simulink model "experiment_file"  (Simulink 8.3)
settings: Solver=ode1  StartTime=0.0  StopTime=inf  FixedStep=0.01  RelTol=1e-3
values from neighbouring files (symbols this model uses):
  accuratepath = interplotation(path)    [Pathplanning.m]    (also in interplotation.m = [accuratepath;interp1([1,insertnum+2],[pathfromstartpoint(i,)
undefined symbols (not defined in the file or in its folder): HIL
libraries: quarc_library x8
settings Model: Creator=drmadill  LastModifiedBy=WXY  SimulationMode=external  ExtModeTrigDuration=1
settings SolverCC: PositivePriorityOrder=on
settings OptimizationCC: ExpressionDepthLimit=2147483647  LifeSpan=auto
settings DebuggingCC: FrameProcessingCompatibilityMsg=error
settings RTWCC: SystemTargetFile=quarc_linux_pi_3.tlc  TemplateMakefile=quarc_linux_pi_3_tmf  Description=QUARC Linux Raspberry Pi 3 Target  ProcessScript=quarc_linux_pi_3_make_rtw_hook
settings STFCustomTargetCC: TargetLibSuffix=.a  TargetPreCompLibLocation=C:\PROGRA~3\QUARC\lib\2017a\LICFC8~1\release  ConcurrentExecutionCompliant=on  SystemTargetFile=quarc_linux_pi_3.tlc
settings GRTTargetCC: TargetLibSuffix=.a  TargetPreCompLibLocation=C:\PROGRA~3\QUARC\lib\2017a\LICFC8~1\release  ParMdlRefBuildCompliant=off  CompOptLevelCompliant=off  GeneratePreprocessorConditionals=Use local settings  MatFileLogging=off  CPPClassGenCompliant=off  ExtMode=on  ExtModeMexFile=quarc_comm  ExtModeMexArgs='-w -d /tmp -uri %u'
settings ConfigComp: CovMetricSettings=dw  CovHtmlReporting=on  CovSaveCumulativeToWorkspaceVar=on  CovSaveSingleToWorkspaceVar=on  CovExternalEMLEnable=off  CovSFcnEnable=off

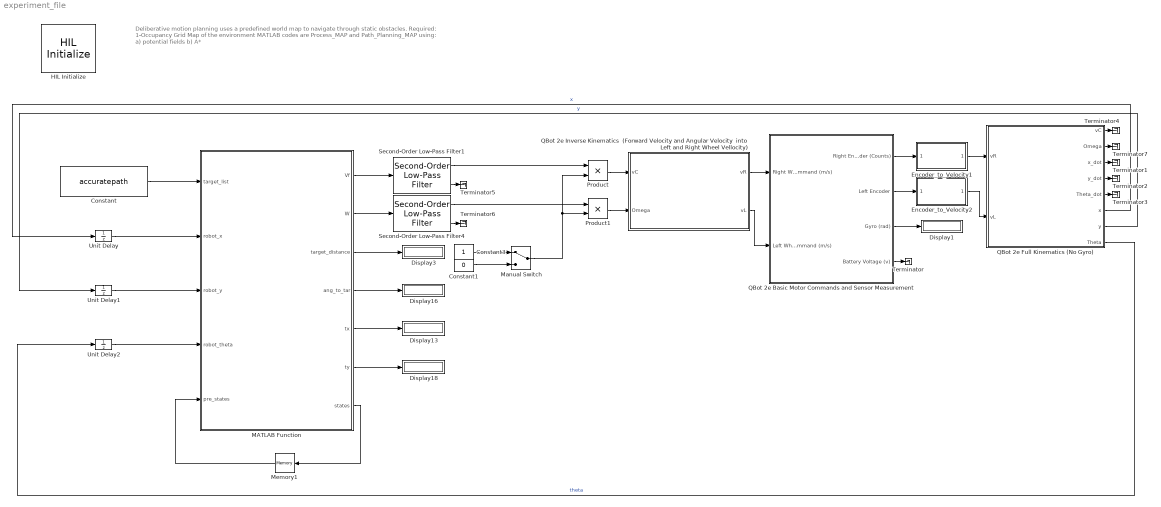
== system experiment_file ==
  note: Deliberative motion planning uses a predefined world map to navigate through static obstacles.
      |
      | Required:
      | 1-Occupancy Grid Map of the environment
      | MATLAB codes are Process_MAP and Path_Planning_MAP using:
      | a) potential fields
      | b) A*
  Constant : Constant  Value=accuratepath
  Constant1 : Constant  Value=0
  Constant3 : Constant
  Display{1,3,13,16,18} (5 alike) : Display
  Encoder_to_Velocity1 : Subsystem
  Encoder_to_Velocity2 : Subsystem
  HIL Initialize : quarc_library/Data Acquisition/Generic/Configuration/HIL Initialize  Priority=-99  object_name=HIL-1  board_type=qbot2e  board_number=0  board_options=pwm0_en=1;pwm0_pin=12;pwm1_en=1;pwm1_pin=13;  exclusive=off  active=off  hardware_clocks=[]  clock_modes=[]  initial_clock_frequencies=[]  set_clock_params_at_start=off  set_clock_params_at_switch_in=off  set_clock_frequencies_at_start=off  set_clock_frequencies_at_switch_in=off  analog_input_channels=[0:5]  analog_input_configurations=[]  analog_input_maximums=[16.5 3.3 3.3 3.3 3.3 3.3]  analog_input_minimums=[0 0 0 0 0 0]  set_analog_input_params_at_start=off  set_analog_input_params_at_switch_in=off  analog_output_channels=[]  analog_output_maximums=[]  analog_output_minimums=[]  initial_analog_outputs=[]  final_analog_outputs=[]  watchdog_analog_outputs=[]  set_analog_output_params_at_start=off  set_analog_output_params_at_switch_in=off  set_analog_outputs_at_start=off  set_analog_outputs_at_switch_in=off  set_analog_outputs_at_terminate=off  set_analog_outputs_at_switch_out=off  set_analog_outputs_on_watchdog=off  digital_input_channels=[28:58]  digital_output_channels=[28:31]  digital_output_configuration=[]  initial_digital_outputs=[0]  final_digital_outputs=[0]  watchdog_digital_outputs=[]  set_digital_output_params_at_start=off  set_digital_output_params_at_switch_in=off  set_digital_outputs_at_start=on  set_digital_outputs_at_switch_in=off  set_digital_outputs_at_terminate=on  set_digital_outputs_at_switch_out=off  set_digital_outputs_on_watchdog=off  encoder_channels=[0:1]  quadrature=[4]  encoder_filter_frequency=[]  initial_encoder_counts=[0]  set_encoder_params_at_start=on  set_encoder_params_at_switch_in=off  set_encoder_counts_at_start=on  set_encoder_counts_at_switch_in=off  pwm_channels=[0:1]  pwm_modes=0  pwm_frequency=100e6 / 4095  pwm_configuration=[0]  pwm_alignment=[0]  pwm_polarity=[1]  pwm_leading_deadband=[]  pwm_trailing_deadband=[]  initial_pwm_outputs=[0]  final_pwm_outputs=[0]  watchdog_pwm_outputs=[]  set_pwm_params_at_start=on  set_pwm_params_at_switch_in=off  set_pwm_outputs_at_start=on  set_pwm_outputs_at_switch_in=off  set_pwm_outputs_at_terminate=on  set_pwm_outputs_at_switch_out=off  set_pwm_outputs_on_watchdog=off  other_output_channels=[2000:2001 14000 16000]  initial_other_outputs=[0 0 0 7]  final_other_outputs=[0 0 0 7]  watchdog_other_outputs=[]  set_other_outputs_at_start=on  set_other_outputs_at_switch_in=off  set_other_outputs_at_terminate=on  set_other_outputs_at_switch_out=off  set_other_outputs_on_watchdog=off
  MATLAB Function : MATLAB Function  TreatAsAtomicUnit=on
  Manual Switch : ManualSwitch
  Memory1 : Memory  X0=[1]
  Product : Product  RndMeth=Zero
  Product1 : Product  RndMeth=Zero
  QBot 2e Basic Motor Commands and Sensor Measurement : Subsystem
  QBot 2e Full Kinematics (No Gyro) : Subsystem
  QBot 2e Inverse Kinematics  (Forward Velocity and Angular Velocity  into Left and Right Wheel Vellocity) : Subsystem
  Second-Order Low-Pass Filter1 : quarc_library/Continuous/Second-Order Low-Pass Filter  params_source=Internal (dialog parameters)  input_width=30  input_zeta=1  input_init=0
  Second-Order Low-Pass Filter4 : quarc_library/Continuous/Second-Order Low-Pass Filter  params_source=Internal (dialog parameters)  input_width=60  input_zeta=1  input_init=0
  Terminator{,1..7} (8 alike) : Terminator
  Unit Delay : UnitDelay  SampleTime=-1
  Unit Delay1 : UnitDelay  SampleTime=-1
  Unit Delay2 : UnitDelay  SampleTime=-1
  wires:
  Constant3/1 -> Manual Switch/1
  Constant1/1 -> Manual Switch/2
  QBot 2e Basic Motor Commands and Sensor Measurement/1(Right Encoder (Counts)) -> Encoder_to_Velocity1/1(Encoder)
  QBot 2e Basic Motor Commands and Sensor Measurement/2(Left Encoder) -> Encoder_to_Velocity2/1(Encoder)
  QBot 2e Basic Motor Commands and Sensor Measurement/3(Gyro (rad)) -> Display1/1
  Encoder_to_Velocity1/1(Velocity) -> QBot 2e Full Kinematics (No Gyro)/1(vR)
  Encoder_to_Velocity2/1(Velocity) -> QBot 2e Full Kinematics (No Gyro)/2(vL)
  Second-Order Low-Pass Filter1/1 -> Product/1
  Second-Order Low-Pass Filter4/1 -> Product1/1
  QBot 2e Inverse Kinematics  (Forward Velocity and Angular Velocity  into Left and Right Wheel Vellocity)/1(vR) -> QBot 2e Basic Motor Commands and Sensor Measurement/1(Right Wheel Command (m/s))
  QBot 2e Inverse Kinematics  (Forward Velocity and Angular Velocity  into Left and Right Wheel Vellocity)/2(vL) -> QBot 2e Basic Motor Commands and Sensor Measurement/2(Left Wheel Command (m/s))
  Product/1 -> QBot 2e Inverse Kinematics  (Forward Velocity and Angular Velocity  into Left and Right Wheel Vellocity)/1(vC)
  Product1/1 -> QBot 2e Inverse Kinematics  (Forward Velocity and Angular Velocity  into Left and Right Wheel Vellocity)/2(Omega)
  Manual Switch/1 -> Product/2, Product1/2
  QBot 2e Full Kinematics (No Gyro)/3(x_dot) -> Terminator1/1
  QBot 2e Full Kinematics (No Gyro)/4(y_dot) -> Terminator2/1
  QBot 2e Full Kinematics (No Gyro)/5(Theta_dot) -> Terminator3/1
  MATLAB Function/3(target_distance) -> Display3/1
  MATLAB Function/4(ang_to_tar) -> Display16/1
  MATLAB Function/1(Vf) -> Second-Order Low-Pass Filter1/1
  MATLAB Function/2(W) -> Second-Order Low-Pass Filter4/1
  QBot 2e Full Kinematics (No Gyro)/8(Theta) -> Unit Delay2/1  "theta"
  MATLAB Function/5(tx) -> Display13/1
  MATLAB Function/6(ty) -> Display18/1
  QBot 2e Full Kinematics (No Gyro)/6(x) -> Unit Delay/1  "x"
  QBot 2e Full Kinematics (No Gyro)/7(y) -> Unit Delay1/1  "y"
  Second-Order Low-Pass Filter1/2 -> Terminator5/1
  Second-Order Low-Pass Filter4/2 -> Terminator6/1
  QBot 2e Full Kinematics (No Gyro)/1(vC) -> Terminator4/1
  QBot 2e Full Kinematics (No Gyro)/2(Omega) -> Terminator7/1
  QBot 2e Basic Motor Commands and Sensor Measurement/4(Battery Voltage (v)) -> Terminator/1
  Constant/1 -> MATLAB Function/1(target_list)
  Unit Delay/1 -> MATLAB Function/2(robot_x)
  Unit Delay1/1 -> MATLAB Function/3(robot_y)
  Unit Delay2/1 -> MATLAB Function/4(robot_theta)
  MATLAB Function/7(states) -> Memory1/1
  Memory1/1 -> MATLAB Function/5(pre_states)

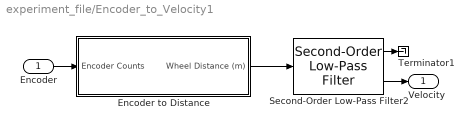
== system experiment_file/Encoder_to_Velocity1 ==
  Encoder : Inport
  Encoder to Distance : Subsystem
  Second-Order Low-Pass Filter2 : quarc_library/Continuous/Second-Order Low-Pass Filter  params_source=Internal (dialog parameters)  input_width=10  input_zeta=1  input_init=0
  Terminator1 : Terminator
  Velocity : Outport
  wires:
  Second-Order Low-Pass Filter2/1 -> Terminator1/1
  Encoder to Distance/1(Wheel Distance (m)) -> Second-Order Low-Pass Filter2/1
  Encoder/1 -> Encoder to Distance/1(Encoder Counts)
  Second-Order Low-Pass Filter2/2 -> Velocity/1

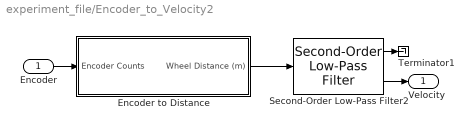
== system experiment_file/Encoder_to_Velocity2 ==
  Encoder : Inport
  Encoder to Distance : Subsystem
  Second-Order Low-Pass Filter2 : quarc_library/Continuous/Second-Order Low-Pass Filter  params_source=Internal (dialog parameters)  input_width=10  input_zeta=1  input_init=0
  Terminator1 : Terminator
  Velocity : Outport
  wires:
  Second-Order Low-Pass Filter2/2 -> Velocity/1
  Encoder/1 -> Encoder to Distance/1(Encoder Counts)
  Encoder to Distance/1(Wheel Distance (m)) -> Second-Order Low-Pass Filter2/1
  Second-Order Low-Pass Filter2/1 -> Terminator1/1

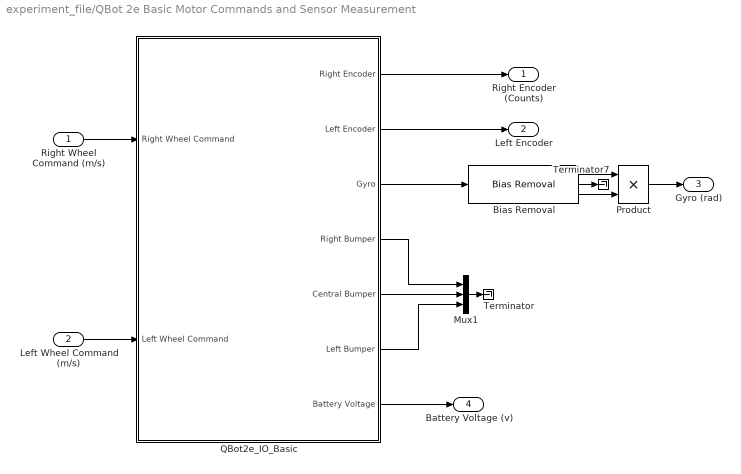
== system experiment_file/QBot 2e Basic Motor Commands and Sensor Measurement ==
  Right Wheel Command (m/s) : Inport
  Left Wheel Command (m/s) : Inport  Port=2
  Bias Removal : quarc_library/Discrete/Bias Removal  start_time=3  end_time=4  switch_id=0  sample_time=qc_get_step_size
      settings: SourceProductName=QUARC Targets
  Mux1 : Mux  Inputs=3
  Product : Product  RndMeth=Zero
  QBot2e_IO_Basic : Subsystem
  Terminator : Terminator
  Terminator7 : Terminator
  Right Encoder (Counts) : Outport
  Left Encoder : Outport  Port=2
  Gyro (rad) : Outport  Port=3
  Battery Voltage (v) : Outport  Port=4
  wires:
  QBot2e_IO_Basic/4(Right Bumper) -> Mux1/1
  QBot2e_IO_Basic/5(Central Bumper) -> Mux1/2
  QBot2e_IO_Basic/6(Left Bumper) -> Mux1/3
  Right Wheel Command (m/s)/1 -> QBot2e_IO_Basic/1(Right Wheel Command)
  Left Wheel Command (m/s)/1 -> QBot2e_IO_Basic/2(Left Wheel Command)
  QBot2e_IO_Basic/1(Right Encoder) -> Right Encoder (Counts)/1
  QBot2e_IO_Basic/2(Left Encoder) -> Left Encoder/1
  QBot2e_IO_Basic/7(Battery Voltage) -> Battery Voltage (v)/1
  Bias Removal/2 -> Terminator7/1
  Bias Removal/1 -> Product/1
  Bias Removal/3 -> Product/2
  Product/1 -> Gyro (rad)/1
  QBot2e_IO_Basic/3(Gyro) -> Bias Removal/1
  Mux1/1 -> Terminator/1

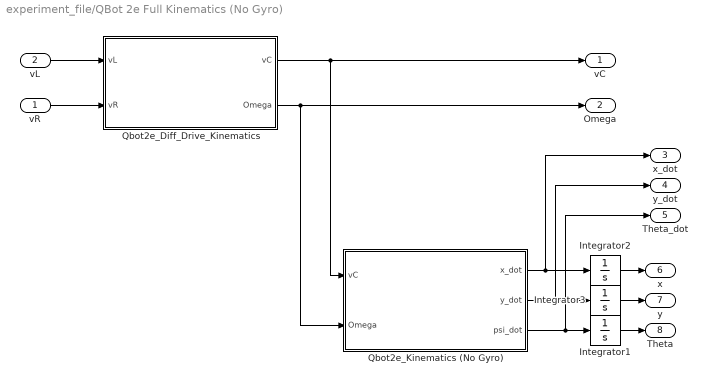
== system experiment_file/QBot 2e Full Kinematics (No Gyro) ==
  vR : Inport
  vL : Inport  Port=2
  Integrator1 : Integrator
  Integrator2 : Integrator
  Integrator3 : Integrator
  Qbot2e_Diff_Drive_Kinematics : Subsystem
  Qbot2e_Kinematics (No Gyro) : Subsystem
  vC : Outport
  Omega : Outport  Port=2
  x_dot : Outport  Port=3
  y_dot : Outport  Port=4
  Theta_dot : Outport  Port=5
  x : Outport  Port=6
  y : Outport  Port=7
  Theta : Outport  Port=8
  wires:
  Integrator1/1 -> Theta/1
  Qbot2e_Kinematics (No Gyro)/3(psi_dot) -> Theta_dot/1, Integrator1/1
  Qbot2e_Kinematics (No Gyro)/1(x_dot) -> x_dot/1, Integrator2/1
  Qbot2e_Kinematics (No Gyro)/2(y_dot) -> y_dot/1, Integrator3/1
  Qbot2e_Diff_Drive_Kinematics/1(vC) -> Qbot2e_Kinematics (No Gyro)/1(vC), vC/1
  vL/1 -> Qbot2e_Diff_Drive_Kinematics/1(vL)
  vR/1 -> Qbot2e_Diff_Drive_Kinematics/2(vR)
  Integrator2/1 -> x/1
  Integrator3/1 -> y/1
  Qbot2e_Diff_Drive_Kinematics/2(Omega) -> Qbot2e_Kinematics (No Gyro)/2(Omega), Omega/1

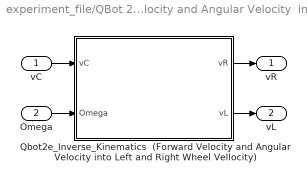
== system experiment_file/QBot 2e Inverse Kinematics  (Forward Velocity and Angular Velocity  into Left and Right Wheel Vellocity) ==
  vC : Inport
  Omega : Inport  Port=2
  Qbot2e_Inverse_Kinematics  (Forward Velocity and Angular Velocity into Left and Right Wheel Vellocity) : MATLAB Function  TreatAsAtomicUnit=on
  vR : Outport
  vL : Outport  Port=2
  wires:
  Qbot2e_Inverse_Kinematics  (Forward Velocity and Angular Velocity into Left and Right Wheel Vellocity)/2(vL) -> vL/1
  Omega/1 -> Qbot2e_Inverse_Kinematics  (Forward Velocity and Angular Velocity into Left and Right Wheel Vellocity)/2(Omega)
  Qbot2e_Inverse_Kinematics  (Forward Velocity and Angular Velocity into Left and Right Wheel Vellocity)/1(vR) -> vR/1
  vC/1 -> Qbot2e_Inverse_Kinematics  (Forward Velocity and Angular Velocity into Left and Right Wheel Vellocity)/1(vC)

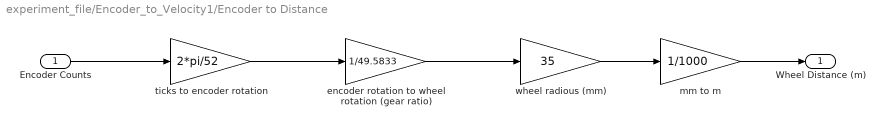
== system experiment_file/Encoder_to_Velocity1/Encoder to Distance ==
  Encoder Counts : Inport
  " encoder rotation to wheel rotation (gear ratio)" : Gain  Gain=1/49.5833
  mm to m : Gain  Gain=1/1000
  ticks to encoder rotation : Gain  Gain=2*pi/52
  wheel radious (mm) : Gain  Gain=35
  Wheel Distance (m) : Outport
  wires:
  Encoder Counts/1 -> ticks to encoder rotation/1
  ticks to encoder rotation/1 -> " encoder rotation to wheel rotation (gear ratio)"/1
  " encoder rotation to wheel rotation (gear ratio)"/1 -> wheel radious (mm)/1
  wheel radious (mm)/1 -> mm to m/1
  mm to m/1 -> Wheel Distance (m)/1

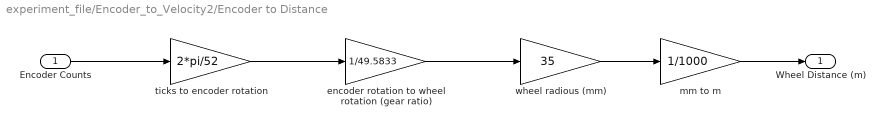
== system experiment_file/Encoder_to_Velocity2/Encoder to Distance ==
  Encoder Counts : Inport
  " encoder rotation to wheel rotation (gear ratio)" : Gain  Gain=1/49.5833
  mm to m : Gain  Gain=1/1000
  ticks to encoder rotation : Gain  Gain=2*pi/52
  wheel radious (mm) : Gain  Gain=35
  Wheel Distance (m) : Outport
  wires:
  mm to m/1 -> Wheel Distance (m)/1
  wheel radious (mm)/1 -> mm to m/1
  " encoder rotation to wheel rotation (gear ratio)"/1 -> wheel radious (mm)/1
  ticks to encoder rotation/1 -> " encoder rotation to wheel rotation (gear ratio)"/1
  Encoder Counts/1 -> ticks to encoder rotation/1

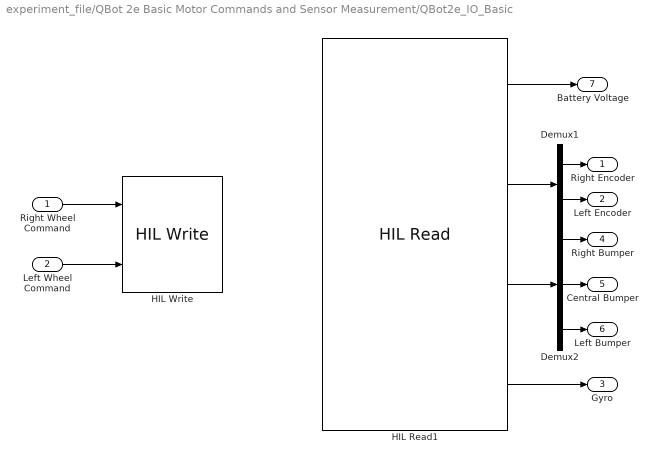
== system experiment_file/QBot 2e Basic Motor Commands and Sensor Measurement/QBot2e_IO_Basic ==
  Right Wheel Command : Inport
  Left Wheel Command : Inport  Port=2
  Demux1 : Demux  Outputs=2
  Demux2 : Demux  Outputs=3
  HIL Read1 : quarc_library/Data Acquisition/Generic/Immediate I//O/HIL Read  object_name=HIL-1  analog_channels=[0]  encoder_channels=[0:1]  digital_channels=[28:30]  other_channels=[1002]  sample_time=qc_get_step_size  active=on  vector_output=on  data_type_mode=Inherit via back propagation  encoder_data_type=double  digital_data_type=boolean
  HIL Write : quarc_library/Data Acquisition/Generic/Immediate I//O/HIL Write  object_name=HIL-1  analog_channels=[]  pwm_channels=[]  digital_channels=[]  other_channels=[2000:2001]  sample_time=-1  active=on  vector_input=off
  Right Encoder : Outport
  Left Encoder : Outport  Port=2
  Gyro : Outport  Port=3
  Right Bumper : Outport  Port=4
  Central Bumper : Outport  Port=5
  Left Bumper : Outport  Port=6
  Battery Voltage : Outport  Port=7
  wires:
  HIL Read1/1 -> Battery Voltage/1
  HIL Read1/3 -> Demux2/1
  HIL Read1/4 -> Gyro/1
  Demux1/1 -> Right Encoder/1
  Demux1/2 -> Left Encoder/1
  Right Wheel Command/1 -> HIL Write/1
  Left Wheel Command/1 -> HIL Write/2
  HIL Read1/2 -> Demux1/1
  Demux2/1 -> Right Bumper/1
  Demux2/2 -> Central Bumper/1
  Demux2/3 -> Left Bumper/1

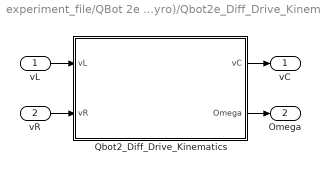
== system experiment_file/QBot 2e Full Kinematics (No Gyro)/Qbot2e_Diff_Drive_Kinematics ==
  vL : Inport
  vR : Inport  Port=2
  Qbot2_Diff_Drive_Kinematics : MATLAB Function  TreatAsAtomicUnit=on
  vC : Outport
  Omega : Outport  Port=2
  wires:
  vL/1 -> Qbot2_Diff_Drive_Kinematics/1(vL)
  Qbot2_Diff_Drive_Kinematics/1(vC) -> vC/1
  vR/1 -> Qbot2_Diff_Drive_Kinematics/2(vR)
  Qbot2_Diff_Drive_Kinematics/2(Omega) -> Omega/1

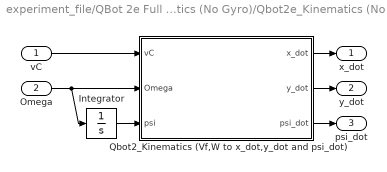
== system experiment_file/QBot 2e Full Kinematics (No Gyro)/Qbot2e_Kinematics (No Gyro) ==
  vC : Inport
  Omega : Inport  Port=2
  Integrator : Integrator
  Qbot2_Kinematics (Vf,W to x_dot,y_dot and psi_dot) : MATLAB Function  TreatAsAtomicUnit=on
  x_dot : Outport
  y_dot : Outport  Port=2
  psi_dot : Outport  Port=3
  wires:
  Qbot2_Kinematics (Vf,W to x_dot,y_dot and psi_dot)/3(psi_dot) -> psi_dot/1
  Integrator/1 -> Qbot2_Kinematics (Vf,W to x_dot,y_dot and psi_dot)/3(psi)
  vC/1 -> Qbot2_Kinematics (Vf,W to x_dot,y_dot and psi_dot)/1(vC)
  Qbot2_Kinematics (Vf,W to x_dot,y_dot and psi_dot)/1(x_dot) -> x_dot/1
  Omega/1 -> Integrator/1, Qbot2_Kinematics (Vf,W to x_dot,y_dot and psi_dot)/2(Omega)
  Qbot2_Kinematics (Vf,W to x_dot,y_dot and psi_dot)/2(y_dot) -> y_dot/1

== matlab function QBot 2e Full Kinematics (No Gyro)/Qbot2e_Diff_Drive_Kinematics/Qbot2_Diff_Drive_Kinematics ==
  data: vL input double; vC output double; vR input double; Omega output double
function [vC,Omega] = fcn(vL,vR)
%#codegen

d= 0.235;

vC=0.5*(vL+vR);
Omega=(1/d)*(vR-vL);

== matlab function QBot 2e Full Kinematics (No Gyro)/Qbot2e_Kinematics (No Gyro)/Qbot2_Kinematics (Vf,W to x_dot,y_dot and psi_dot) ==
  data: vC input double; x_dot output double; Omega input double; y_dot output double; psi input double; psi_dot output double
function [x_dot,y_dot,psi_dot] = fcn(vC,Omega,psi)
%#codegen


x_dot=cos(psi)*vC;
y_dot=sin(psi)*vC;
psi_dot= Omega;

== matlab function MATLAB Function ==
  data: target_list input double; Vf output double; robot_x input double; robot_y input double; robot_theta input double; pre_states input double; W output double; target_distance output double; ang_to_tar output double; tx output double; ty output double; states output double
function [Vf, W, target_distance, ang_to_tar, tx, ty, states] = ...
    WaypointControl(target_list, robot_x,robot_y,robot_theta, pre_states)
vlimit = 0.5; %最大限速
dist_thr = 0.1;
ang_thr = 10*pi/180;
method = 1;
step=1;
%step = 3; % 预估目标点的间隔
stop = 10;

%%%只需要改Kv_1 Kw_1就好
Kv_1 = 2; % 左轮速度常数   目标v=kv*x
Kw_1 = 1; % 左轮转角速度常数  目标w=kw*x

Kv_2 = 0.2;
Kw_2 = 0.9;
Psi_d = pi; % 机器人最终停止时角度（朝向）

% 初始化输出参数
 Vf=0;
 W=0;
 target_distance=0;
 ang_to_tar=0;
 finished_path_flag=0; 
 
 persistent Vf_1 end_flag;
 
 if isempty(Vf_1)
     Vf_1=0;
 end
 if isempty(end_flag)
    end_flag = 0;
 end
 
 %储存上一次的状态信息
states = pre_states;

rx =robot_x;
ry = robot_y;
rtheta = check_angle(robot_theta); %限定转角在 [-pi ,pi]之间


target_xy = [rx ry];  %当前坐标x y
[n xy] = size(target_list);  % n代表有n个点; xy=2
if n==2 && xy==1
    target_xy = [target_list(1,1) target_list(2,1)];
    n = 1;
else
    for i=1:n  %遍历所有规划的点
        if states(1) == i  %找到前面的规划点
            for j=1:xy
                if i < n-stop  %预瞄
                    target_xy(j) = target_list(i+stop, j);
                else
                    target_xy(j) = target_list(i, j);
                end
            end
        end
    end
end

tx = target_xy(1);
ty = target_xy(2);
target_distance = find_dist(rx, ry, tx, ty);
ang_to_tar= find_theta(rx, ry, rtheta, tx, ty);

if ((states(1) == n) && (target_distance <= dist_thr))  %到达终点或离终点

        Vf=0;
        W=0;
        
       if (end_flag == 1) && (target_distance <= dist_thr) % 最终到达目的地时朝向转到要求位置
            [Vf, W] = ClosedLoop_Sequential(0, check_angle(check_angle(Psi_d)-check_angle(rtheta)), vlimit, ang_thr, dist_thr, Kv_1, Kw_1, Vf_1); 
             Vf_1=Vf;
       end
   
else
    % 已经到达了目标点附近
    if (target_distance <= dist_thr) && (end_flag==0)
            states(1) = pre_states(1) + step;%1;
          if( pre_states(1) > 0 )      
             while (abs((target_list(states(1),1))-(target_list(pre_states(1),1)))<2*dist_thr) && (abs((target_list(states(1),2))-(target_list(pre_states(1),2)))<2*dist_thr)
                 if (states(1)<=(n-step))
                     states(1) = states(1) + step;%1;
                 else
                     states(1)=n;
                 end
             end
          else
              states(1)=states(1)+step;
          end
     
          %防止数组越界
         if states(1) >= n 
            states(1) = n;
            end_flag=1;  %停车
         end

    else
        if method == 2
            [Vf, W] = ClosedLoop_Both(target_distance,  ang_to_tar, vlimit, Kv_2, Kw_2);    
        else
            [Vf, W] = ClosedLoop_Sequential(target_distance,  ang_to_tar, vlimit, ang_thr, dist_thr, Kv_1, Kw_1, Vf_1); 
            Vf_1=Vf;
        end       
    end
    
end

return;

% 认为机器人转角应在-180到180度之间
function [y] = check_angle(x)
y = x;
while ( x > pi || x < -pi)
    if x > pi
        y = x - 2*pi;
    else
        y = x + 2*pi;
    end
end
return;

% 目标点与当前点距离
function dist = find_dist(rx, ry, tx, ty)
dist = sqrt((rx-tx)^2 + (ry-ty)^2);
return;

% 机器人当前需要转过的角度
function [theta]= find_theta(rx, ry, rtheta, tx, ty)

X = tx - rx;
Y = ty - ry;
theta = atan2(Y, X);
theta = check_angle(check_angle(theta)-check_angle(rtheta));

return;

% 根据目标距离和转角算出机器人的前进速度和转角速度
function [Vf, W] = ClosedLoop_Both(dist, theta, vlimit, Kv,Kw)

d = 0.23;
vmax = vlimit;
wmax = (2*vmax);
W = Kw*theta;

Vf = Kv * dist;

w_sign = sign(W); % 保留转角符号
if abs(W) > wmax
    W = w_sign*wmax;
end
if abs(Vf)> vlimit
    Vf = sign(Vf)*vlimit;%%%%% Vf = abs(Vf)*vlimit;
end

return;

% 仅前进或仅转弯
function [Vf, W] = ClosedLoop_Sequential(dist, theta, vlimit, ang_thr, dist_thr, Kv, Kw, Vf_1)

d = 0.23;
vmax = vlimit;
wmax = (2*vmax);

if (((abs(theta) > ang_thr))  && (Vf_1<0.01)) || (abs(theta) > 5*ang_thr) 
        W=Kw*theta;
        Vf=0;
        if abs(W)> wmax
            W=sign(W)*wmax;
        end
else
        Vf=Kv*dist;
       
        if abs(Vf)>vlimit
            Vf=sign(Vf)*vlimit;
        end
        
        W=0;
        
end
return;

== matlab function QBot 2e Inverse Kinematics (Forward Velocity and Angular Velocity into Left and Right Wheel Vellocity)/Qbot2e_Inverse_Kinematics (Forward Velocity and Angular Velocity into Left and Right Wheel Vellocity) ==
  data: vR output double; vL output double; vC input double; Omega input double
function [vR,vL] = fcn(vC , Omega)
%#codegen

d=0.235; 
% Eqn Based on the eqn 4.52 (W is the angular velocity)

vR = vC + Omega*d/2;
vL= vC - Omega*d/2;
